simulink model "testMagnetoField"  (R2021a)
settings: Solver=VariableStepAuto  StartTime=0.0  StopTime=Torb  RelTol=1e-3
settings Model: DataDictionary=databus.sldd  Creator=Laura  LastModifiedBy=Laura

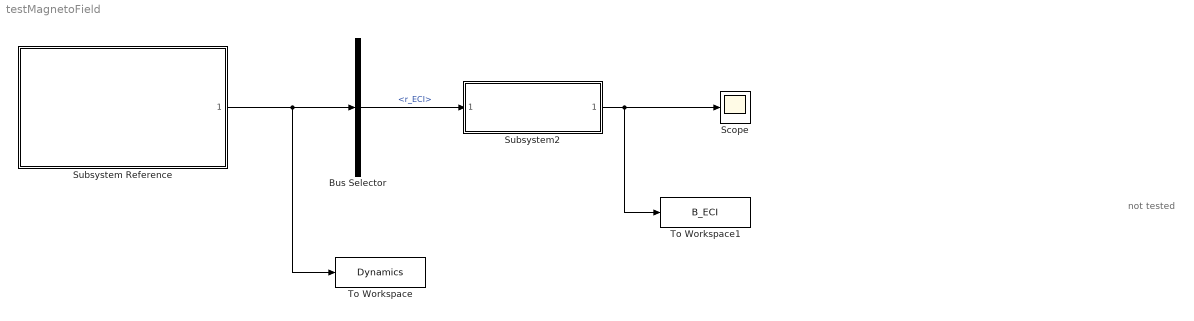
== system testMagnetoField ==
  note: not tested
  Bus Selector : BusSelector  OutputSignals=r_ECI
  Scope : Scope
  Subsystem Reference : Subsystem  ReferencedSubsystem=SCDynamics
  Subsystem2 : Subsystem  ReferencedSubsystem=MagDipole
  To Workspace : ToWorkspace  VariableName=Dynamics  SaveFormat=Timeseries  SampleTime=-1
  To Workspace1 : ToWorkspace  VariableName=B_ECI  SaveFormat=Timeseries  SampleTime=-1
  wires:
  Subsystem2/1 -> To Workspace1/1, Scope/1
  Subsystem Reference/1 -> To Workspace/1, Bus Selector/1
  Bus Selector/1 -> Subsystem2/1  "<r_ECI>"
